simulink model "step_responses"  (R2016b)
settings: Solver=VariableStepAuto  StartTime=0.0  StopTime=10.0  RelTol=1e-3
undefined symbols (not defined in the file): den, dendi, num, numdi, ts
settings Model: Creator=AdrianCortez  LastModifiedBy=AdrianCortez
settings DataIOCC: ReturnWorkspaceOutputs=on
settings DebuggingCC: UnconnectedInputMsg=none  UnconnectedOutputMsg=none  UnconnectedLineMsg=none
settings ModelReferenceCC: EnableRefExpFcnMdlSchedulingChecks=off
settings SFSimCC: SimUseLocalCustomCode=on
settings RTWCC: RTWUseLocalCustomCode=on

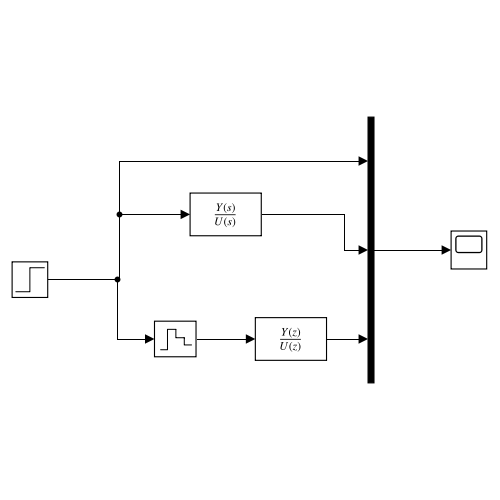
[thumbnail: Simulink's stored preview of the top-level diagram]
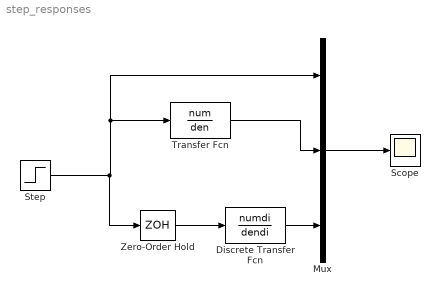
== system step_responses ==
  Discrete Transfer Fcn : DiscreteTransferFcn  Numerator=numdi  Denominator=dendi
  Mux : Mux  Inputs=3
  Scope : Scope
  Step : Step  SampleTime=0
  Transfer Fcn : TransferFcn  Numerator=num  Denominator=den
  Zero-Order Hold : ZeroOrderHold  SampleTime=ts
  wires:
  Step/1 -> Zero-Order Hold/1, Mux/1, Transfer Fcn/1
  Transfer Fcn/1 -> Mux/2
  Discrete Transfer Fcn/1 -> Mux/3
  Mux/1 -> Scope/1
  Zero-Order Hold/1 -> Discrete Transfer Fcn/1
